simulink model "Example_MATLAB"  (R2017b)
settings: Solver=VariableStepAuto  StartTime=0.0  StopTime=10.0  RelTol=1e-3
settings Model: Creator=LunkP  LastModifiedBy=LunkP

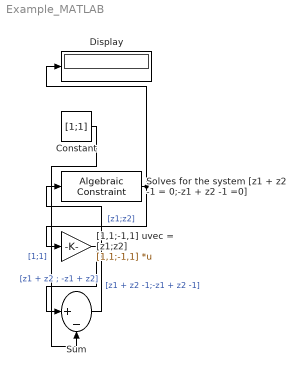
== system Example_MATLAB ==
  Constant : Constant  Value=[1;1]  VectorParams1D=off
  Display : Display
  Solves for the system [z1 + z2 -1 = 0;-z1 + z2 -1 =0] : AlgebraicConstraint  InitialGuess=[0;1]
  Sum : Sum  Inputs=|+-
  "[1,1;-1,1] uvec = [z1;z2]" : Gain  Gain=[1,1;-1,1]  Multiplication=Matrix(K*u) (u vector)
  wires:
  Constant/1 -> Sum/2  "[1;1]"
  Solves for the system [z1 + z2 -1 = 0;-z1 + z2 -1 =0]/1 -> Display/1, "[1,1;-1,1] uvec = [z1;z2]"/1  "[z1;z2]"
  Sum/1 -> Solves for the system [z1 + z2 -1 = 0;-z1 + z2 -1 =0]/1  "[z1 + z2 -1;-z1 + z2 -1]"
  "[1,1;-1,1] uvec = [z1;z2]"/1 -> Sum/1  "[z1 + z2 ; -z1 + z2]"
